simulink model "FrameBaseSignal"  (R2022b)
settings: Solver=VariableStepAuto  StartTime=0.0  StopTime=10.0  RelTol=1e-3
undefined symbols (not defined in the file): CarrierTs, CodeTs, Delay, Dimension, f_chirp_max, f_chirp_min, gcbh, rcfiltgaincompat, T_chirp, Ts
libraries: commdigbbndam3 x1, commfilt2 x1, simulink x1
settings Model: Creator=79327  LastModifiedBy=79327

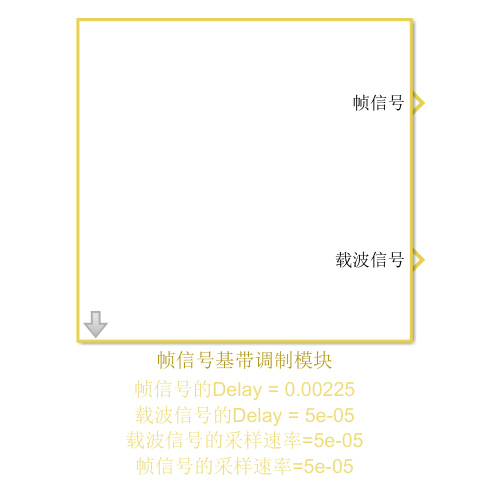
[thumbnail: Simulink's stored preview of the top-level diagram]
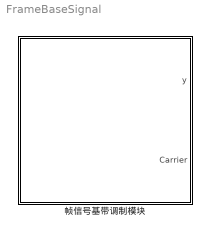
== system FrameBaseSignal ==
  帧信号基带调制模块 : Subsystem  TreatAsAtomicUnit=on  mask{OutputSize=1000, CodeTs=CodeTs, CarrierTs=CarrierTs, N=round(CodeTs/CarrierTs), Coding_Element=[0 3 1 2 3 2 1 3].', Delay_Frame=0.00225, Delay_Carrier=5e-05, T_Frame=5e-05, T_Carrier=5e-05}
      mask prompts: OutputSize "输出信号维度"; CodeTs "采样时间"; CarrierTs "载波采样时间"; N "输出信号维度"; Coding_Element "帧信号编码码元(Coding_Element)"; Delay_Frame "帧信号的延时(单位s)"; Delay_Carrier "载波信号的延时"; T_Frame "帧信号的采样时间"; T_Carrier "载波信号的采样时间"
      mask init:
      | modelpath = gcb; %获得当前模块的路径
      |             modelhandle = gcbh;    %获得当前模块的句柄
      |             buffer12 = getSimulinkBlockHandle([modelpath,'/Buffer12'],true);
      |             filter = getSimulinkBlockHandle([modelpath,'/Raised Cosine Transmit Filter'],true);
      |             
      |             %计算buffer12产生的时延
      |             N = eval(get_param(modelhandle,'N'));
      |             bufer12_outputsize = eval(get_param(buffer12,'N'));
      |             buffer12_f = str2double(get_param(filter,'N'));
      |             BufferDelay = bufer12_outputsize * CodeTs / buffer12_f;        
      |             
      |             %计算filter产生的时延
      |             filter_span = str2double(get_param(filter,'filtSpan'));
      |             filterDelay = filter_span * CodeTs / 2;
      | 
      |             %设置帧信号的时延
      |             set_param(modelhandle,'Delay_Frame',num2str(BufferDelay + filterDelay));
      |             %设置载波信号的时延
      |             set_param(modelhandle,'Delay_Carrier',num2str(N * CarrierTs));
      |             %设置帧信号的采样时间
      |             set_param(modelhandle,'T_Carrier',num2str(CodeTs));
      |             %设置载波信号的采样时间
      |             set_param(modelhandle,'T_Frame',num2str(CodeTs));
      settings: AttributesFormatString=|
      | 帧信号的Delay = %<Delay_Frame>
      | 载波信号的Delay = %<Delay_Carrier>
      | 载波信号的采样速率=%<T_Carrier>
      | 帧信号的采样速率=%<T_Frame>
      mask DialogControl ParameterGroupVar Prompt: 参数
      mask DialogControl Container3 Prompt: 输出信号延时(与0时刻相比)
      mask DialogControl Container5 Prompt: 输出信号采样时间

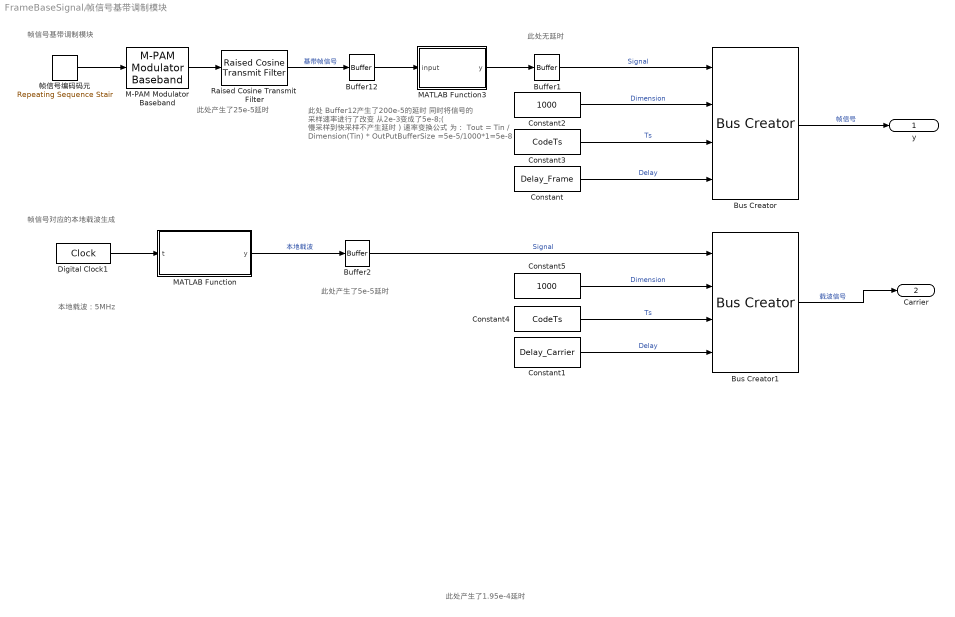
== system FrameBaseSignal/帧信号基带调制模块 ==
  note: 帧信号基带调制模块
  note: 此处产生了25e-5延时
  note: 此处无延时
  note: 此处产生了1.95e-4延时
  note: 本地载波：5MHz
  note: 此处产生了5e-5延时
  note: 帧信号对应的本地载波生成
  note: 此处 Buffer12产生了200e-5的延时
      | 同时将信号的 采样速率进行了改变
      | 从2e-3变成了5e-8;( 慢采样到快采样不产生延时 )
      | 速率变换公式 为：
      | Tout = Tin / Dimension(Tin) * OutPutBufferSize
      | =5e-5/1000*1=5e-8
  Buffer1 : Buffer  N=N  OutputFrames=off
  Buffer12 : Buffer  N=4 * N  OutputFrames=off
  Buffer2 : Buffer  N=N  OutputFrames=off
      settings: AttributesFormatString=Delay = %<N> * CarrierTs
  Bus Creator : BusCreator  Inputs=Signal,Dimension,Ts,Delay  OutDataTypeStr=Bus: SignalBus1  NonVirtualBus=on
  Bus Creator1 : BusCreator  Inputs=Signal,Dimension,Ts,Delay  OutDataTypeStr=Bus: SignalBus1  NonVirtualBus=on
  Constant : Constant  Value=Delay_Frame  SampleTime=CodeTs
  Constant1 : Constant  Value=Delay_Carrier  SampleTime=CodeTs
  Constant2 : Constant  Value=1000  SampleTime=CodeTs
  Constant3 : Constant  Value=CodeTs  SampleTime=CodeTs
  Constant4 : Constant  Value=CodeTs  SampleTime=-1
  Constant5 : Constant  Value=1000  SampleTime=CodeTs
  Digital Clock1 : DigitalClock  SampleTime=CarrierTs
      settings: AttributesFormatString=|
      | CarrierTs = %<SampleTime>
      | CarruerFreq = 1 / CarrierTs
  M-PAM Modulator Baseband : commdigbbndam3/M-PAM Modulator Baseband  M=4  InType=Integer  Enc=Gray  PowType=Min. distance between symbols  MinDist=2  AvgPow=1  PeakPow=1  outDtype=double  outWordLen=16  outUDDataType=sfix(16)  outFracLenMode=Best precision  outFracLen=15  outDataTypeStr=double  outLastDataTypeStr=double
  MATLAB Function : MATLAB Function  InitFcn=|  TreatAsAtomicUnit=on
      | f_chirp_min=4.8e6;
      | f_chirp_max=5.2e6;
      | T_chirp=4e-4;
  MATLAB Function3 : MATLAB Function  TreatAsAtomicUnit=on
  Raised Cosine Transmit Filter : commfilt2/Raised Cosine Transmit Filter  filtType=Square root  R=0.25  filtSpan=10  N=100  filterGain=rcfiltgaincompat(gcbh)  InputProcessing=Columns as channels (frame based)  RateOptions=Enforce single-rate processing  framing=Mute  checkCoeff=off  variableName=rcTxFilt  checkGain=Normalized  sampMode=Mute  saveAsFlag=0  currentFiltSpan=10  D=(10)/2  launchFVT=on  roundingMode=Floor  overflowMode=off  coeffDataTypeStr=Inherit: Same word length as input  coeffMin=[]  coeffMax=[]  coeffLastDataTypeStr=Inherit: Same word length as input  outputDataTypeStr=Inherit: Same as accumulator  outputMin=[]  outputMax=[]  outputLastDataTypeStr=Inherit: Same as accumulator
  帧信号编码码元 : simulink/Sources/Repeating Sequence Stair  OutValues=Coding_Element  tsamp=CodeTs  OutMin=[]  OutMax=[]  OutDataTypeStr=double  OutputDataTypeScalingMode=double  OutDataType=fixdt(0,8)  ConRadixGroup=Best Precision: Vector-wise  OutScaling=2^-12
      settings: AttributesFormatString=|
      | 帧信号编码码元 = %<OutValues>
      | 采样时间 = %<tsamp>
  y : Outport  OutDataTypeStr=Bus: SignalBus1
  Carrier : Outport  Port=2  OutDataTypeStr=Bus: SignalBus1
  wires:
  帧信号编码码元/1 -> M-PAM Modulator Baseband/1
  M-PAM Modulator Baseband/1 -> Raised Cosine Transmit Filter/1
  Raised Cosine Transmit Filter/1 -> Buffer12/1  "基带帧信号"
  MATLAB Function3/1(y) -> Buffer1/1
  Buffer12/1 -> MATLAB Function3/1(input)
  Digital Clock1/1 -> MATLAB Function/1(t)
  MATLAB Function/1(y) -> Buffer2/1  "本地载波"
  Buffer1/1 -> Bus Creator/1  "Signal"
  Constant/1 -> Bus Creator/4  "Delay"
  Bus Creator/1 -> y/1  "帧信号"
  Buffer2/1 -> Bus Creator1/1  "Signal"
  Constant1/1 -> Bus Creator1/4  "Delay"
  Bus Creator1/1 -> Carrier/1  "载波信号"
  Constant2/1 -> Bus Creator/2  "Dimension"
  Constant3/1 -> Bus Creator/3  "Ts"
  Constant5/1 -> Bus Creator1/2  "Dimension"
  Constant4/1 -> Bus Creator1/3  "Ts"

== matlab function FrameBaseSignal/帧信号基带调制模块/MATLAB Function ==
  data: y output; t input; f_chirp_min parameter; f_chirp_max parameter; T_chirp parameter
% function y = carrierGenerator(t)
%     fc = 5e6;
%     y = exp(1i*2*pi*fc*t);

function y = carrierGenerator(t, f_chirp_min, f_chirp_max, T_chirp)
    k_chirp = (f_chirp_max-f_chirp_min)/T_chirp;
    t = mod(t,T_chirp);
    y = exp(1i*2*pi*(f_chirp_min*t+0.5*k_chirp*t^2));

end

== matlab function FrameBaseSignal/帧信号基带调制模块/MATLAB Function3 ==
  data: y output; input input
% function y = carrierGenerator(t)
%     fc = 5e6;
%     y = exp(1i*2*pi*fc*t);

function y = rateTransition(input)
    p = 10;
    q = 1;
    y = resample(input,p,q);
%     y(1:100) = repmat(y(100),1,100);
%     y(end-99:end) = repmat(y(end-99),1,100);
end
